simulink library "realisticSensorProcessing_cl"  (R2020a)
settings: Solver=VariableStepAuto  StartTime=0.0  StopTime=10.0  RelTol=1e-3
undefined symbols (not defined in the file or in its folder): initializeBussesFromBlock
settings Model: Creator=mcobb  LastModifiedBy=Zak
settings DataIOCC: ReturnWorkspaceOutputs=off
settings DebuggingCC: ArithmeticOperatorsInVariantConditions=warning
settings SFSimCC: CustomCodeUndefinedFunction=UseInterfaceOnly

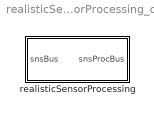
== system realisticSensorProcessing_cl ==
  realisticSensorProcessing : Subsystem  LoadFcn=initializeBussesFromBlock(gcb)  InitFcn=initializeBussesFromBlock(gcb)  StartFcn=initializeBussesFromBlock(gcb)

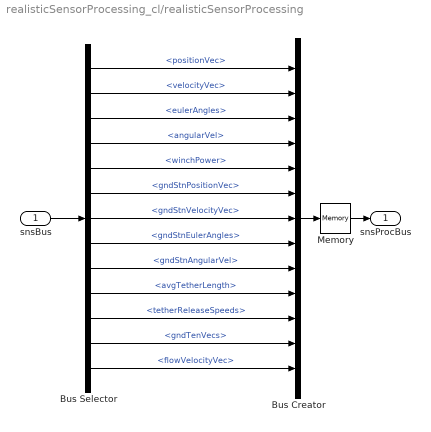
== system realisticSensorProcessing_cl/realisticSensorProcessing ==
  snsBus : Inport  OutDataTypeStr=Bus: sensorsBus
  Bus Creator : BusCreator  Inputs=13  OutDataTypeStr=Bus: sensorsProcessingBus  NonVirtualBus=on
  Bus Selector : BusSelector  OutputSignals=positionVec,velocityVec,eulerAngles,angularVel,winchPower,gndStnPositionVec,gndStnVelocityVec,gndStnEulerAngles,gndStnAngularVel,avgTetherLength,tetherReleaseSpeeds,gndTenVecs,flowVelocityVec
  Memory : Memory
  snsProcBus : Outport  OutDataTypeStr=Bus: sensorsProcessingBus  VectorParamsAs1DForOutWhenUnconnected=off
  wires:
  Bus Selector/3 -> Bus Creator/3  "<eulerAngles>"
  Bus Selector/12 -> Bus Creator/12  "<gndTenVecs>"
  Bus Selector/10 -> Bus Creator/10  "<avgTetherLength>"
  Bus Selector/8 -> Bus Creator/8  "<gndStnEulerAngles>"
  Bus Selector/13 -> Bus Creator/13  "<flowVelocityVec>"
  Bus Selector/2 -> Bus Creator/2  "<velocityVec>"
  Bus Selector/6 -> Bus Creator/6  "<gndStnPositionVec>"
  Bus Selector/4 -> Bus Creator/4  "<angularVel>"
  Bus Selector/1 -> Bus Creator/1  "<positionVec>"
  Bus Selector/5 -> Bus Creator/5  "<winchPower>"
  snsBus/1 -> Bus Selector/1
  Bus Selector/7 -> Bus Creator/7  "<gndStnVelocityVec>"
  Bus Selector/11 -> Bus Creator/11  "<tetherReleaseSpeeds>"
  Bus Creator/1 -> Memory/1
  Bus Selector/9 -> Bus Creator/9  "<gndStnAngularVel>"
  Memory/1 -> snsProcBus/1
